simulink library "commdigbbndtcm2"  (Simulink 6.0)
settings: Solver=ode45  SolverMode=SingleTasking  StartTime=0.0  StopTime=10.0  RelTol=1e-3
undefined symbols (not defined in the file or in its folder): constpts, cplxconstpts, D, j, Mnum
libraries: commutil2 x3, dspsigattribs x3, commcnvcod2 x3, commdigbbndam2 x2
settings Model: Creator=ashivapr  LastModifiedBy=cvora  ExtModeAutoUpdateStatusClock=off  ProdHWDeviceType=Specified
settings DataIOCC: SignalLoggingName=logsOut
settings OptimizationCC: BooleanDataType=off
settings DebuggingCC: CheckExecutionContextPreStartOutputMsg=on  CheckExecutionContextRuntimeOutputMsg=on  SolverPrmCheckMsg=none
settings HardwareCC: ProdHWDeviceType=Specified  TargetUnknown=on
settings SFSimCC: SFSimApplyToAllLibs=on  SFSimBuildMode=Incremental

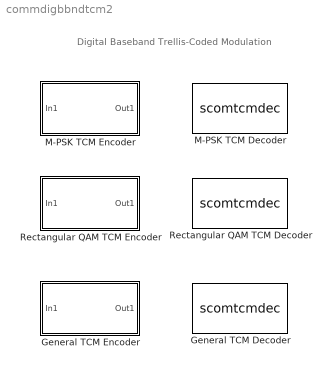
== system commdigbbndtcm2 ==
  note: Digital Baseband
      | Trellis-Coded Modulation
  General TCM Decoder : S-Function  FunctionName=scomtcmdec  Parameters=t.k,t.n,t.numStates,t.outputs,t.nextStates, real(cplxconstpts), imag(cplxconstpts), tbdepth, opmode, reset  SFunctionModules=viterbi_acs_tbdec  mask(General TCM Decoder){trellis=poly2trellis([1 3],[1 0 0; 0 5 2]), constpts=exp(2*pi*j*[0 4 2 6 1 5 3 7]/8), tbdepth=21, opmode=Continuous, reset=off}
      mask prompts: trellis "Trellis structure:"; constpts "Signal constellation:"; tbdepth "Traceback depth:"; opmode "Operation mode:"; reset "Enable the reset input port"
      mask help:
      | Use the Viterbi algorithm to decode trellis-coded modulation data, mapped using the Signal constellation parameter that expects complex constellation points in the set-partitioned order.
      |
      | The Trellis structure parameter must be a valid MATLAB trellis structure. To check if a structure is a valid trellis structure, use the istrellis function in MATLAB.
      mask init:
      | [e, s, cplxconstpts, t] = commblkgentcmdec(gcb,'init');
      | if ~isempty(e.msg)
      | 	error(e.msg); 
      | end
      mask Help: helpview(commbhelp)
      mask StyleString: edit,edit,edit,popup(Continuous|Truncated|Terminated),checkbox
      mask CallbackString: |||commblkgentcmdec(gcb,'cbOpmode');|
      mask Display:
      | disp('General\nTCM');
      | port_label('input',s.ports.i1,s.ports.i1s);
      | port_label('input',s.ports.i2,s.ports.i2s);
      | port_label('output',s.ports.o1,s.ports.o1s);
  General TCM Encoder : Subsystem  PropExecContextAcrossSSBoundary=on  mask(General TCM Encoder){trellis=poly2trellis([1 3],[1 0 0; 0 5 2]), constpts=exp(2*pi*j*[0 4 2 6 1 5 3 7]/8)}
      mask prompts: trellis "Trellis structure:"; constpts "Signal constellation:"
      mask help:
      | Convolutionally encode binary data and perform signal mapping using the Signal constellation parameter, which expects complex constellation points in the set-partitioned order.
      |
      | The Trellis structure parameter must be a valid MATLAB trellis structure. To check if a structure is a valid trellis structure, use the istrellis function in MATLAB.
      mask init:
      | [constpts Mnum err] = commblkgentcmenc(gcb);
      | if ~isempty(err.msg)
      | 	error(err.msg);
      | end
      mask Help: helpview(commbhelp)
      mask Display: disp('General\nTCM')
  M-PSK TCM Decoder : S-Function  FunctionName=scomtcmdec  Parameters=t.k,t.n,t.numStates,t.outputs,t.nextStates, real(cplxconstpts), imag(cplxconstpts), tbdepth, opmode, reset  SFunctionModules=viterbi_acs_tbdec  mask(M-PSK TCM Decoder){trellis=poly2trellis([1 3],[1 0 0; 0 5 2]), M=8, tbdepth=21, opmode=Continuous, reset=off}
      mask prompts: trellis "Trellis structure:"; M "M-ary number:"; tbdepth "Traceback depth:"; opmode "Operation mode:"; reset "Enable the reset input port"
      mask help: Uses the Viterbi algorithm to decode TCM data for PSK modulated signal.
      mask init:
      | [e, s, cplxconstpts, t] = commblkpsktcmdec(gcb,'init');
      | if ~isempty(e.msg)
      | 	error(e.msg); 
      | end
      mask Help: helpview(commbhelp)
      mask StyleString: edit,popup(4|8|16),edit,popup(Continuous|Truncated|Terminated),checkbox
      mask CallbackString: |||commblkpsktcmdec(gcb,'cbOpmode');|
      mask Display:
      | disp('M-PSK\nTCM');
      | port_label('input',s.ports.i1,s.ports.i1s);
      | port_label('input',s.ports.i2,s.ports.i2s);
      | port_label('output',s.ports.o1,s.ports.o1s);
  M-PSK TCM Encoder : Subsystem  PropExecContextAcrossSSBoundary=on  mask(M-PSK TCM Encoder ){trellis=poly2trellis([1 3],[1 0 0; 0 5 2]), M=8}
      mask prompts: trellis "Trellis structure:"; M "M-ary number:"
      mask help:
      | Convolutionally encode binary data and modulate using the phase shift keying method.
      |
      | The Trellis structure parameter must be a valid MATLAB trellis structure. To check if a structure is a valid trellis structure, use the istrellis function in MATLAB.
      mask init:
      | [constpts Mnum err] = commblkpsktcmenc(gcb);
      | if ~isempty(err.msg)
      | 	error(err.msg);
      | end
      mask Help: helpview(commbhelp)
      mask StyleString: edit,popup(4|8|16)
      mask Display: disp('M-PSK\nTCM')
  Rectangular QAM TCM Decoder : S-Function  FunctionName=scomtcmdec  Parameters=t.k,t.n,t.numStates,t.outputs,t.nextStates, real(cplxconstpts), imag(cplxconstpts), tbdepth, opmode, reset  SFunctionModules=viterbi_acs_tbdec  mask(Rectangular QAM TCM Decoder){trellis=poly2trellis([3 1 1], [ 5 2 0 0; 0 0 1 0; 0 0 0 1]), M=16, tbdepth=21, opmode=Continuous, reset=off}
      mask prompts: trellis "Trellis structure:"; M "M-ary number:"; tbdepth "Traceback depth:"; opmode "Operation mode:"; reset "Enable the reset input port"
      mask help:
      | Use the Viterbi algorithm to decode trellis-coded modulation data, modulated using the quadrature amplitude modulation method.
      |
      | The Trellis structure parameter must be a valid MATLAB trellis structure. To check if a structure is a valid trellis structure, use the istrellis function in MATLAB.
      mask init:
      | [e, s, cplxconstpts, t] = commblkqamtcmdec(gcb,'init');
      | if ~isempty(e.msg)
      | 	error(e.msg); 
      | end
      mask Help: helpview(commbhelp)
      mask StyleString: edit,popup(4|8|16|32|64),edit,popup(Continuous|Truncated|Terminated),checkbox
      mask CallbackString: |||commblkqamtcmdec(gcb,'cbOpmode');|
      mask Display:
      | disp('Rectangular\nQAM TCM');
      | port_label('input',s.ports.i1,s.ports.i1s);
      | port_label('input',s.ports.i2,s.ports.i2s);
      | port_label('output',s.ports.o1,s.ports.o1s);
  Rectangular QAM TCM Encoder : Subsystem  PropExecContextAcrossSSBoundary=on  mask(Rectangular QAM TCM Encoder){trellis=poly2trellis([3 1 1], [ 5 2 0 0; 0 0 1 0; 0 0 0 1]), M=16}
      mask prompts: trellis "Trellis structure:"; M "M-ary number:"
      mask help:
      | Convolutionally encode binary data and modulate using the quadrature amplitude modulation method.
      |
      | The Trellis structure parameter must be a valid MATLAB trellis structure. To check if a structure is a valid trellis structure, use the istrellis function in MATLAB.
      mask init:
      | [constpts Mnum err] = commblkqamtcmenc(gcb);
      | if ~isempty(err.msg)
      | 	error(err.msg);
      | end
      mask Help: helpview(commbhelp)
      mask StyleString: edit,popup(4|8|16|32|64)
      mask Display: disp('Rectangular\nQAM TCM')

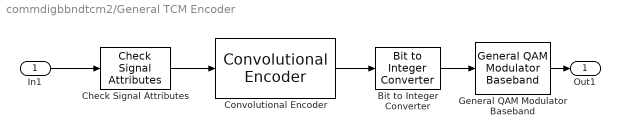
== system commdigbbndtcm2/General TCM Encoder ==
  In1 : Inport  LatchInput=off
  Bit to Integer Converter : commutil2/Bit to Integer Converter  nbits=log2(Mnum)
  Check Signal Attributes : dspsigattribs/Check Signal Attributes  SigAttribCheckMethod=Matches attributes exactly  Complexity=Ignore  Frame=Sample-based  DimsCheckMethod=Ignore  Dimensions=1-D  DatatypeCheckMethod=Ignore  DatatypeGeneral=Boolean  DtypeFloatSpecific=Any floating-point  DtypeFixedSpecific=Any fixed-point  DtypeIntSpecific=Any integer  SampleMode=Ignore
  Convolutional Encoder : commcnvcod2/Convolutional Encoder  trellis=trellis  reset=None
  General QAM Modulator Baseband : commdigbbndam2/General QAM Modulator Baseband  SigCon=constpts  numSamp=1
  Out1 : Outport
  wires:
  General QAM Modulator Baseband/1 -> Out1/1
  Convolutional Encoder/1 -> Bit to Integer Converter/1
  In1/1 -> Check Signal Attributes/1
  Bit to Integer Converter/1 -> General QAM Modulator Baseband/1
  Check Signal Attributes/1 -> Convolutional Encoder/1

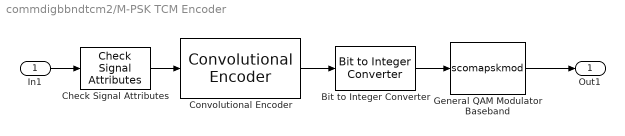
== system commdigbbndtcm2/M-PSK TCM Encoder ==
  In1 : Inport  LatchInput=off
  Bit to Integer Converter : commutil2/Bit to Integer Converter  nbits=log2(Mnum)
  Check Signal Attributes : dspsigattribs/Check Signal Attributes  SigAttribCheckMethod=Matches attributes exactly  Complexity=Ignore  Frame=Sample-based  DimsCheckMethod=Ignore  Dimensions=1-D  DatatypeCheckMethod=Ignore  DatatypeGeneral=Boolean  DtypeFloatSpecific=Any floating-point  DtypeFixedSpecific=Any fixed-point  DtypeIntSpecific=Any integer  SampleMode=Ignore
  Convolutional Encoder : commcnvcod2/Convolutional Encoder  trellis=trellis  reset=None
  General QAM Modulator Baseband : S-Function  AncestorBlock=|  FunctionName=scomapskmod  Parameters=4,2,1,1,1,1,1,0,numSamp,SigConRe,SigConIm,5  mask(General QAM Modulator Baseband){SigCon=constpts, numSamp=1}
      | commdigbbndam2/General QAM
      | Modulator
      | Baseband
      mask prompts: SigCon "Signal constellation:"; numSamp "Samples per symbol:"
      mask help:
      | Modulate the input signal using the quadrature amplitude modulation method.
      |
      | The block only accepts integers as input. For sample-based integer input, the input must be a scalar. For frame-based integer input, the input must be a column vector.
      |
      | In case of frame-based input, the width of the output frame equals the product of the number of symbols and the Samples per symbol value.
      |
      | In case of sample-based input, the output sample time equals the symbol period divided by the Samples per symbol value.
      mask init:
      | SigConRe=real(SigCon);
      | SigConIm=imag(SigCon);
      mask Help: helpview(commbhelp)
      mask Display:
      | plot(0,0,100,100,[5+15*[0 1 1 2 2 3] 50 50 50 50+1.5*[[0:.8:10] [10:1.6:20] [20:.8:30]]],[85+8*[1 1 -1 -1 1 1] 85 99 75 85+10*[sin([0:.8:10]*pi*2/5) sin([10:1.6:20]*pi/5) sin([20:.8:30]*pi*2/5)]]);
      | disp('\nGeneral\nQAM')
  Out1 : Outport
  wires:
  Bit to Integer Converter/1 -> General QAM Modulator Baseband/1
  General QAM Modulator Baseband/1 -> Out1/1
  Convolutional Encoder/1 -> Bit to Integer Converter/1
  In1/1 -> Check Signal Attributes/1
  Check Signal Attributes/1 -> Convolutional Encoder/1

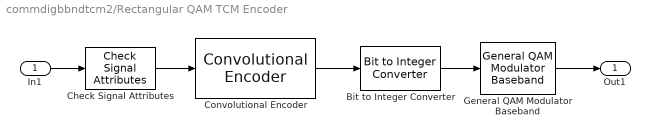
== system commdigbbndtcm2/Rectangular QAM TCM Encoder ==
  In1 : Inport  LatchInput=off
  Bit to Integer Converter : commutil2/Bit to Integer Converter  nbits=log2(Mnum)
  Check Signal Attributes : dspsigattribs/Check Signal Attributes  SigAttribCheckMethod=Matches attributes exactly  Complexity=Ignore  Frame=Sample-based  DimsCheckMethod=Ignore  Dimensions=1-D  DatatypeCheckMethod=Ignore  DatatypeGeneral=Boolean  DtypeFloatSpecific=Any floating-point  DtypeFixedSpecific=Any fixed-point  DtypeIntSpecific=Any integer  SampleMode=Ignore
  Convolutional Encoder : commcnvcod2/Convolutional Encoder  trellis=trellis  reset=None
  General QAM Modulator Baseband : commdigbbndam2/General QAM Modulator Baseband  SigCon=constpts  numSamp=1
  Out1 : Outport
  wires:
  Bit to Integer Converter/1 -> General QAM Modulator Baseband/1
  In1/1 -> Check Signal Attributes/1
  Convolutional Encoder/1 -> Bit to Integer Converter/1
  General QAM Modulator Baseband/1 -> Out1/1
  Check Signal Attributes/1 -> Convolutional Encoder/1
